simulink model "Nonlinear_heli_model"  (R2018a)
settings: Solver=VariableStepAuto  StartTime=0.0  StopTime=10.0  RelTol=1e-3
values from neighbouring files (symbols this model uses):
  B_p = 0.01325    [heli_parameters.m]
  B_y = 0.8513    [heli_parameters.m]
  F_cpp = 1    [heli_parameters.m]
  F_cpy = 1    [heli_parameters.m]
  F_cyp = 1    [heli_parameters.m]
  F_cyy = 1    [heli_parameters.m]
  g = 9.81    [Spoustec_simu.m]    (also in heli_parameters.m)
  h = 0.00714    [Spoustec_simu.m]    (also in heli_parameters.m)
  J_eqp = 0.0332    [heli_parameters.m]
  J_eqy = 0.0371    [heli_parameters.m]
  K_pp = 0.02638    [heli_parameters.m]
  K_py = 0.00189    [heli_parameters.m]
  K_yp = 0.002096    [heli_parameters.m]
  K_yy = 0.01871    [heli_parameters.m]
  l_mc = 0.0122    [heli_parameters.m]
  m = 1.3872    [Spoustec_simu.m]    (also in heli_parameters.m)
  psi_0 = 0    [heli_parameters.m]
  theta_0 = -0.7853981634    [heli_parameters.m]
libraries: mpclib x3, cstblocks x2
settings Model: Creator=ja  LastModifiedBy=ja

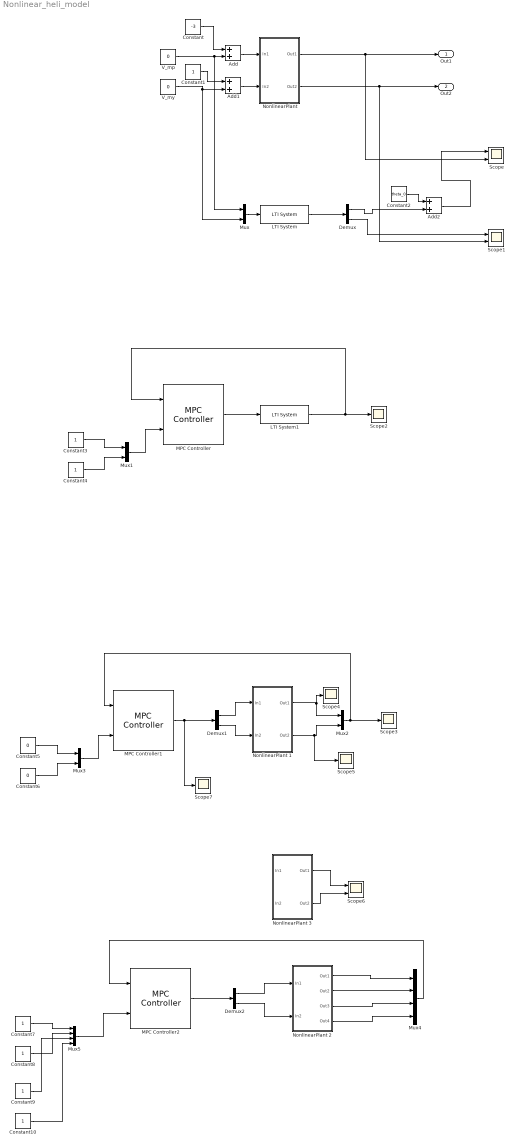
== system Nonlinear_heli_model ==
  Add : Sum
  Add1 : Sum
  Add2 : Sum
  Constant : Constant  Value=-3
  Constant{1,3..4,7..10} (7 alike) : Constant
  Constant2 : Constant  Value=theta_0
  Constant5 : Constant  Value=0
  Constant6 : Constant  Value=0
  Demux : Demux  Outputs=2
  Demux1 : Demux  Outputs=2
  Demux2 : Demux  Outputs=2
  LTI System : cstblocks/LTI System  sys=LinearPlant  IC=[]
  LTI System1 : cstblocks/LTI System  sys=LinearPlant  IC=[]
  MPC Controller : mpclib/MPC Controller  SCDEnableBlockLinearizationSpecification=on  mpcobj=mpc1  is_multiple=0  enable_value=0  return_u0=off  updateMPCinCallerWorkspace=on  ref_from_ws=off  ref_signal_name=[]  ref_preview=off  md_from_ws=off  md_signal_name=[]  md_preview=off  from_project=off  project_file=MPCtask.mat  md_inport=off  mv_inport=off  cost_outport=off  return_sequence=off  return_qpstatus=off  return_state=off  state_inport=off  lims_inport=off  cc_inport=off  ywt_inport=off  is_designfromscratch=0  uwt_inport=off  duwt_inport=off  rhoeps_inport=off  uref_inport=off  n_ts=0.01  n_p=50  n_mv=2  n_md=0  n_ud=0  n_mo=2  n_uo=0  BlockDataType=double  SampleTimeInherited=off  switch_inport=off
  MPC Controller1 : mpclib/MPC Controller  SCDEnableBlockLinearizationSpecification=on  mpcobj=mpc1  is_multiple=0  enable_value=0  return_u0=off  updateMPCinCallerWorkspace=on  ref_from_ws=off  ref_signal_name=[]  ref_preview=off  md_from_ws=off  md_signal_name=[]  md_preview=off  from_project=off  project_file=MPCtask.mat  md_inport=off  mv_inport=off  cost_outport=off  return_sequence=off  return_qpstatus=off  return_state=off  state_inport=off  lims_inport=off  cc_inport=off  ywt_inport=off  is_designfromscratch=0  uwt_inport=off  duwt_inport=off  rhoeps_inport=off  uref_inport=off  n_ts=0.01  n_p=50  n_mv=2  n_md=0  n_ud=0  n_mo=2  n_uo=0  BlockDataType=double  SampleTimeInherited=off  switch_inport=off
  MPC Controller2 : mpclib/MPC Controller  SCDEnableBlockLinearizationSpecification=on  is_multiple=0  enable_value=0  return_u0=off  updateMPCinCallerWorkspace=on  ref_from_ws=off  ref_signal_name=[]  ref_preview=off  md_from_ws=off  md_signal_name=[]  md_preview=off  from_project=off  project_file=MPCtask.mat  md_inport=off  mv_inport=off  cost_outport=off  return_sequence=off  return_qpstatus=off  return_state=off  state_inport=off  lims_inport=off  cc_inport=off  ywt_inport=off  is_designfromscratch=0  uwt_inport=off  duwt_inport=off  rhoeps_inport=off  uref_inport=off  n_ts=0.1  n_p=10  n_mv=2  n_md=0  n_ud=0  n_mo=4  n_uo=0  BlockDataType=double  SampleTimeInherited=off  switch_inport=off
  Mux{,1..3} (4 alike) : Mux  Inputs=2
  Mux4 : Mux
  Mux5 : Mux
  "NonlinearPlant " : Subsystem
  NonlinearPlant 1 : Subsystem
  NonlinearPlant 2 : Subsystem
  NonlinearPlant 3 : Subsystem
  Scope : Scope  NumInputPorts=2
  Scope1 : Scope  NumInputPorts=2
  Scope{2..5,7} (5 alike) : Scope
  Scope6 : Scope  NumInputPorts=2
  "V_mp " : Constant  Value=0
  V_my : Constant  Value=0
  Out1 : Outport
  Out2 : Outport  Port=2
  wires:
  "V_mp "/1 -> Add/2, Mux/1
  V_my/1 -> Add1/2, Mux/2
  "NonlinearPlant "/1(Out1) -> Scope/2, Out1/1
  "NonlinearPlant "/2(Out2) -> Scope1/2, Out2/1
  Mux/1 -> LTI System/1
  LTI System/1 -> Demux/1
  Demux/1 -> Add2/2
  Demux/2 -> Scope1/1
  Constant/1 -> Add/1
  Add/1 -> "NonlinearPlant "/1(In1)
  Add1/1 -> "NonlinearPlant "/2(In2)
  Constant1/1 -> Add1/1
  Constant2/1 -> Add2/1
  Add2/1 -> Scope/1
  MPC Controller/1 -> LTI System1/1
  LTI System1/1 -> Scope2/1, MPC Controller/1
  Mux1/1 -> MPC Controller/2
  Constant3/1 -> Mux1/1
  Constant4/1 -> Mux1/2
  MPC Controller1/1 -> Scope7/1, Demux1/1
  Demux1/1 -> NonlinearPlant 1/1(In1)
  Demux1/2 -> NonlinearPlant 1/2(In2)
  NonlinearPlant 1/1(Out1) -> Scope4/1, Mux2/1
  NonlinearPlant 1/2(Out2) -> Scope5/1, Mux2/2
  Mux2/1 -> MPC Controller1/1, Scope3/1
  Constant6/1 -> Mux3/2
  Constant5/1 -> Mux3/1
  Mux3/1 -> MPC Controller1/2
  MPC Controller2/1 -> Demux2/1
  Demux2/2 -> NonlinearPlant 2/2(In2)
  Demux2/1 -> NonlinearPlant 2/1(In1)
  NonlinearPlant 2/1(Out1) -> Mux4/1
  NonlinearPlant 2/2(Out2) -> Mux4/2
  NonlinearPlant 2/3(Out3) -> Mux4/3
  NonlinearPlant 2/4(Out4) -> Mux4/4
  Mux4/1 -> MPC Controller2/1
  Constant8/1 -> Mux5/2
  Constant7/1 -> Mux5/1
  Mux5/1 -> MPC Controller2/2
  Constant10/1 -> Mux5/4
  Constant9/1 -> Mux5/3
  NonlinearPlant 3/1(Out1) -> Scope6/1
  NonlinearPlant 3/2(Out2) -> Scope6/2

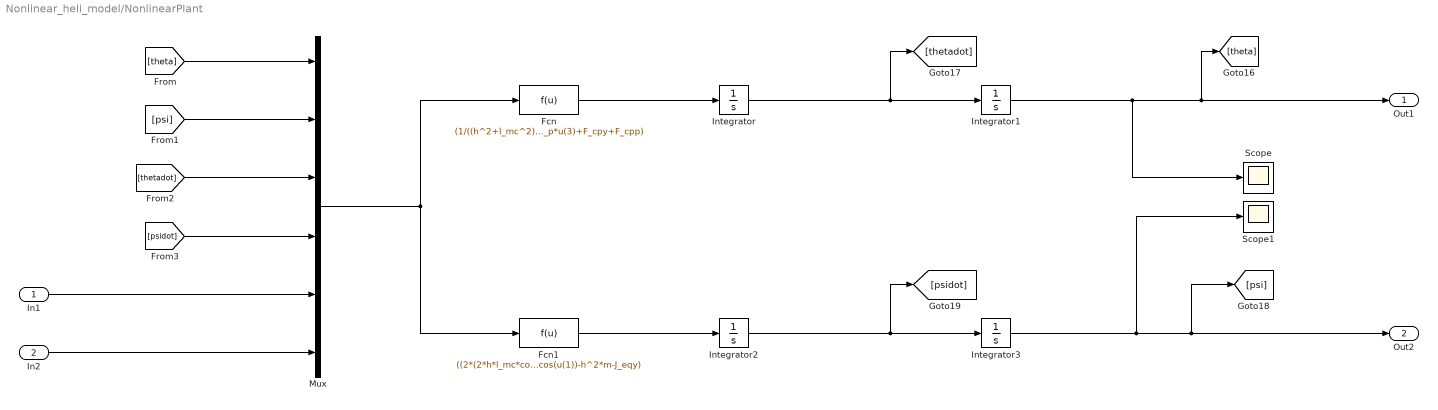
== system Nonlinear_heli_model/NonlinearPlant  ==
  In1 : Inport
  In2 : Inport  Port=2
  Fcn : Fcn  Expr=(1/((h^2+l_mc^2)*m+J_eqp))*(2*m*(h*l_mc*cos(u(1))^2+sin(u(1))*(h^2/2-l_mc^2/2)*cos(u(1))-(h*l_mc)/2)*u(4)^2-cos(u(1))*g*l_mc*m-sin(u(1))*g*h*m+K_pp*u(5)+K_py*u(6)-B_p*u(3)+F_cpy+F_cpp)
  Fcn1 : Fcn  Expr=((2*(2*h*l_mc*cos(u(1))^2+sin(u(1))*(h^2-l_mc^2)*cos(u(1))-h*l_mc)*m*u(3)+B_y)*u(4)-cos(u(1))*(K_yy*u(6)+K_yp*u(5)+F_cyp+F_cyy))/(m*(h^2-l_mc^2)*cos(u(1))^2-2*sin(u(1))*h*m*l_mc*cos(u(1))-h^2*m-J_eqy)
  Integrator : Integrator
  Integrator1 : Integrator  InitialCondition=-0.7853981634
  Integrator2 : Integrator
  Integrator3 : Integrator
  Mux : Mux  Inputs=6
  Scope : Scope
  Scope1 : Scope
  Out1 : Outport
  Out2 : Outport  Port=2
  wires:
  [psi] -> Mux/2
  Fcn/1 -> Integrator/1
  In1/1 -> Mux/5
  Mux/1 -> Fcn1/1, Fcn/1
  [thetadot] -> Mux/3
  Integrator2/1 -> [psidot], Integrator3/1
  Integrator3/1 -> Scope1/1, Out2/1, [psi]
  Fcn1/1 -> Integrator2/1
  In2/1 -> Mux/6
  [theta] -> Mux/1
  Integrator/1 -> [thetadot], Integrator1/1
  Integrator1/1 -> Scope/1, Out1/1, [theta]
  [psidot] -> Mux/4

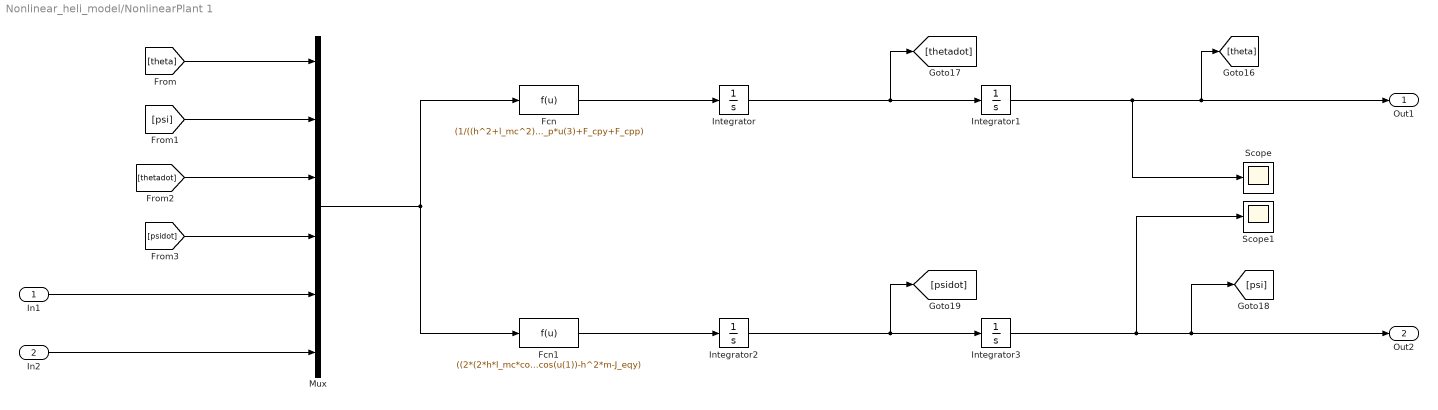
== system Nonlinear_heli_model/NonlinearPlant 1 ==
  In1 : Inport
  In2 : Inport  Port=2
  Fcn : Fcn  Expr=(1/((h^2+l_mc^2)*m+J_eqp))*(2*m*(h*l_mc*cos(u(1))^2+sin(u(1))*(h^2/2-l_mc^2/2)*cos(u(1))-(h*l_mc)/2)*u(4)^2-cos(u(1))*g*l_mc*m-sin(u(1))*g*h*m+K_pp*u(5)+K_py*u(6)-B_p*u(3)+F_cpy+F_cpp)
  Fcn1 : Fcn  Expr=((2*(2*h*l_mc*cos(u(1))^2+sin(u(1))*(h^2-l_mc^2)*cos(u(1))-h*l_mc)*m*u(3)+B_y)*u(4)-cos(u(1))*(K_yy*u(6)+K_yp*u(5)+F_cyp+F_cyy))/(m*(h^2-l_mc^2)*cos(u(1))^2-2*sin(u(1))*h*m*l_mc*cos(u(1))-h^2*m-J_eqy)
  Integrator : Integrator
  Integrator1 : Integrator  InitialCondition=-0.7853981634
  Integrator2 : Integrator
  Integrator3 : Integrator
  Mux : Mux  Inputs=6
  Scope : Scope
  Scope1 : Scope
  Out1 : Outport
  Out2 : Outport  Port=2
  wires:
  [psi] -> Mux/2
  Fcn/1 -> Integrator/1
  In1/1 -> Mux/5
  Mux/1 -> Fcn1/1, Fcn/1
  [thetadot] -> Mux/3
  Integrator2/1 -> [psidot], Integrator3/1
  Integrator3/1 -> Scope1/1, Out2/1, [psi]
  Fcn1/1 -> Integrator2/1
  In2/1 -> Mux/6
  [theta] -> Mux/1
  Integrator/1 -> [thetadot], Integrator1/1
  Integrator1/1 -> Scope/1, Out1/1, [theta]
  [psidot] -> Mux/4

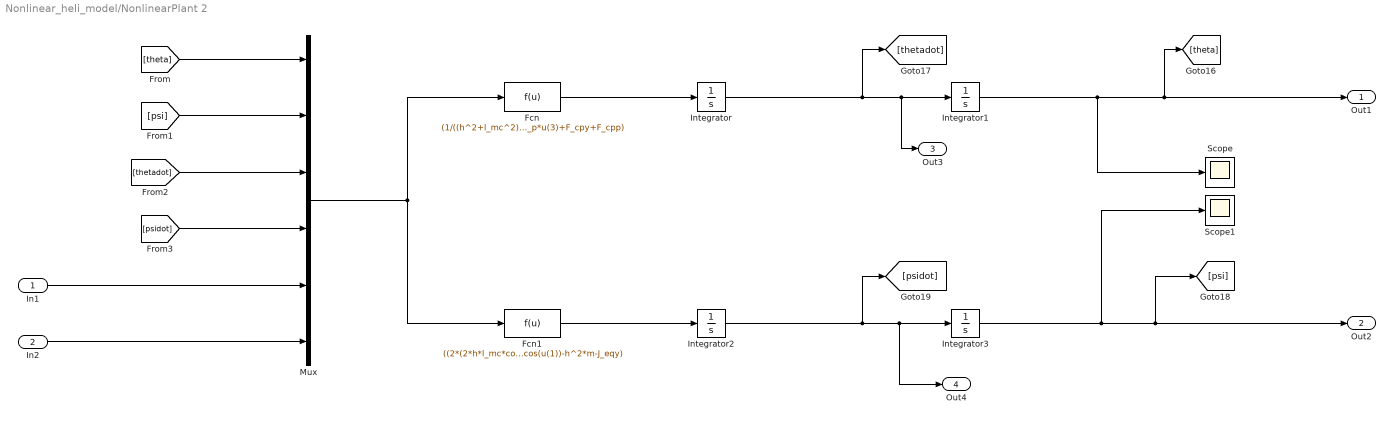
== system Nonlinear_heli_model/NonlinearPlant 2 ==
  In1 : Inport
  In2 : Inport  Port=2
  Fcn : Fcn  Expr=(1/((h^2+l_mc^2)*m+J_eqp))*(2*m*(h*l_mc*cos(u(1))^2+sin(u(1))*(h^2/2-l_mc^2/2)*cos(u(1))-(h*l_mc)/2)*u(4)^2-cos(u(1))*g*l_mc*m-sin(u(1))*g*h*m+K_pp*u(5)+K_py*u(6)-B_p*u(3)+F_cpy+F_cpp)
  Fcn1 : Fcn  Expr=((2*(2*h*l_mc*cos(u(1))^2+sin(u(1))*(h^2-l_mc^2)*cos(u(1))-h*l_mc)*m*u(3)+B_y)*u(4)-cos(u(1))*(K_yy*u(6)+K_yp*u(5)+F_cyp+F_cyy))/(m*(h^2-l_mc^2)*cos(u(1))^2-2*sin(u(1))*h*m*l_mc*cos(u(1))-h^2*m-J_eqy)
  Integrator : Integrator
  Integrator1 : Integrator  InitialCondition=-0.7853981634
  Integrator2 : Integrator
  Integrator3 : Integrator
  Mux : Mux  Inputs=6
  Scope : Scope
  Scope1 : Scope
  Out1 : Outport
  Out2 : Outport  Port=2
  Out3 : Outport  Port=3
  Out4 : Outport  Port=4
  wires:
  [psi] -> Mux/2
  Fcn/1 -> Integrator/1
  In1/1 -> Mux/5
  Mux/1 -> Fcn1/1, Fcn/1
  [thetadot] -> Mux/3
  Integrator2/1 -> [psidot], Out4/1, Integrator3/1
  Integrator3/1 -> Scope1/1, Out2/1, [psi]
  Fcn1/1 -> Integrator2/1
  In2/1 -> Mux/6
  [theta] -> Mux/1
  Integrator/1 -> [thetadot], Out3/1, Integrator1/1
  Integrator1/1 -> Scope/1, Out1/1, [theta]
  [psidot] -> Mux/4

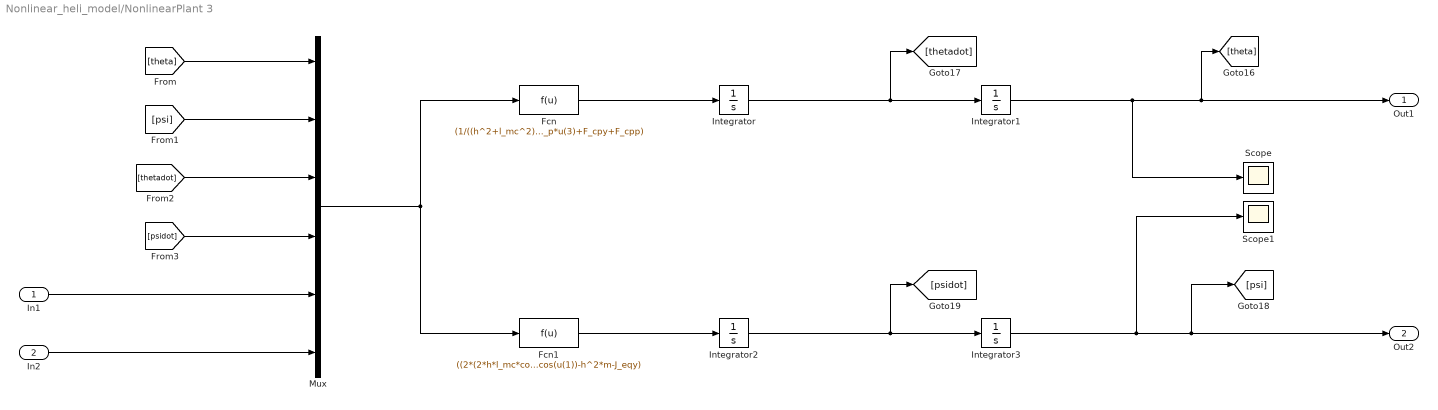
== system Nonlinear_heli_model/NonlinearPlant 3 ==
  In1 : Inport
  In2 : Inport  Port=2
  Fcn : Fcn  Expr=(1/((h^2+l_mc^2)*m+J_eqp))*(2*m*(h*l_mc*cos(u(1))^2+sin(u(1))*(h^2/2-l_mc^2/2)*cos(u(1))-(h*l_mc)/2)*u(4)^2-cos(u(1))*g*l_mc*m-sin(u(1))*g*h*m+K_pp*u(5)+K_py*u(6)-B_p*u(3)+F_cpy+F_cpp)
  Fcn1 : Fcn  Expr=((2*(2*h*l_mc*cos(u(1))^2+sin(u(1))*(h^2-l_mc^2)*cos(u(1))-h*l_mc)*m*u(3)+B_y)*u(4)-cos(u(1))*(K_yy*u(6)+K_yp*u(5)+F_cyp+F_cyy))/(m*(h^2-l_mc^2)*cos(u(1))^2-2*sin(u(1))*h*m*l_mc*cos(u(1))-h^2*m-J_eqy)
  Integrator : Integrator
  Integrator1 : Integrator  InitialCondition=theta_0
  Integrator2 : Integrator
  Integrator3 : Integrator  InitialCondition=psi_0
  Mux : Mux  Inputs=6
  Scope : Scope
  Scope1 : Scope
  Out1 : Outport
  Out2 : Outport  Port=2
  wires:
  [psi] -> Mux/2
  Fcn/1 -> Integrator/1
  In1/1 -> Mux/5
  Mux/1 -> Fcn1/1, Fcn/1
  [thetadot] -> Mux/3
  Integrator2/1 -> [psidot], Integrator3/1
  Integrator3/1 -> Scope1/1, Out2/1, [psi]
  Fcn1/1 -> Integrator2/1
  In2/1 -> Mux/6
  [theta] -> Mux/1
  Integrator/1 -> [thetadot], Integrator1/1
  Integrator1/1 -> Scope/1, Out1/1, [theta]
  [psidot] -> Mux/4
